simulink model "sim"  (R2018a)
settings: Solver=VariableStepAuto  StartTime=0.0  StopTime=10.0  RelTol=1e-3
values from neighbouring files (symbols this model uses):
  g = 9.8    [cod.m]
settings Model: Creator=daniel  LastModifiedBy=daniel

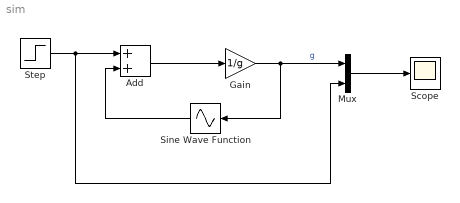
== system sim ==
  Add : Sum
  Gain : Gain  Gain=1/g
  Mux : Mux  Inputs=2
  Scope : Scope
  Sine Wave Function : Sin  TimeSource=Use external signal  SampleTime=0
  Step : Step  SampleTime=0
  wires:
  Step/1 -> Mux/2, Add/1
  Add/1 -> Gain/1
  Gain/1 -> Mux/1, Sine Wave Function/1  "g"
  Sine Wave Function/1 -> Add/2
  Mux/1 -> Scope/1
